simulink model "P2_son"  (R2021b)
settings: Solver=VariableStepAuto  StartTime=0.0  StopTime=10.0  RelTol=1e-3
undefined symbols (not defined in the file or in its folder): k, sample_time
libraries: simulink x1
settings Model: Creator=11639  LastModifiedBy=11639

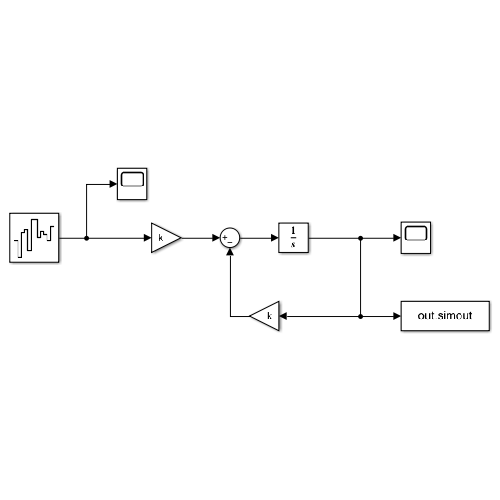
[thumbnail: Simulink's stored preview of the top-level diagram]
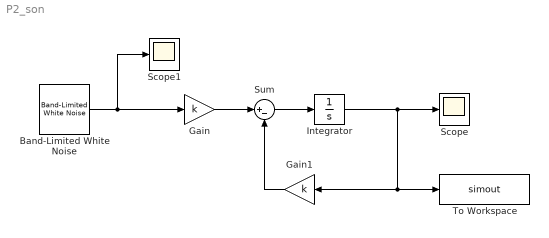
== system P2_son ==
  Band-Limited White Noise : simulink/Sources/Band-Limited White Noise  Cov=noise_power  Ts=sample_time  seed=seed
  Gain : Gain  Gain=k
  Gain1 : Gain  Gain=k
  Integrator : Integrator
  Scope : Scope
  Scope1 : Scope
  Sum : Sum  Inputs=|+-
  To Workspace : ToWorkspace  VariableName=simout  SaveFormat=Timeseries  SampleTime=-1
  wires:
  Band-Limited White Noise/1 -> Scope1/1, Gain/1
  Gain1/1 -> Sum/2
  Gain/1 -> Sum/1
  Sum/1 -> Integrator/1
  Integrator/1 -> To Workspace/1, Gain1/1, Scope/1
